simulink model "PI2GDL"  (R2018a)
settings: Solver=VariableStepAuto  StartTime=0.0  StopTime=200  RelTol=1e-3
values from neighbouring files (symbols this model uses):
  B = (T*tc)/(Ti)    (= 0.482939903103)    [Controlador2GDL.m]    (also in Examen2.m)
  k = 9.22    [Controlador2GDL.m]    (also in ControladorAlfaroPI1GDL_ControlEstricto.m; ControladorAlfaroPI1GDL_ControlSuave.m; Examen2.m)
  Kp = (a)/(k*(tc+to).^2)    [Controlador2GDL.m]    (also in ControladorAlfaroPI1GDL_ControlEstricto.m = 0.669122125129; ControladorAlfaroPI1GDL_ControlSuave.m = 0.469559386056; Examen2.m)
  L = 3.17    [Controlador2GDL.m]    (also in ControladorAlfaroPI1GDL_ControlEstricto.m; ControladorAlfaroPI1GDL_ControlSuave.m; Examen2.m)
  T = 34.31    [Controlador2GDL.m]    (also in ControladorAlfaroPI1GDL_ControlEstricto.m; ControladorAlfaroPI1GDL_ControlSuave.m; Examen2.m)
  Ti = T*(a/(1+to))    (= 14.2088072572)    [Controlador2GDL.m]    (also in ControladorAlfaroPI1GDL_ControlEstricto.m = 0.0291460215681; ControladorAlfaroPI1GDL_ControlSuave.m = 0.0291460215681; Examen2.m)
  Ts = 0.1    [Examen2.m]
settings Model: Creator=Rafael  LastModifiedBy=wivill
settings CodeAppCC: StateflowObjectComments=on

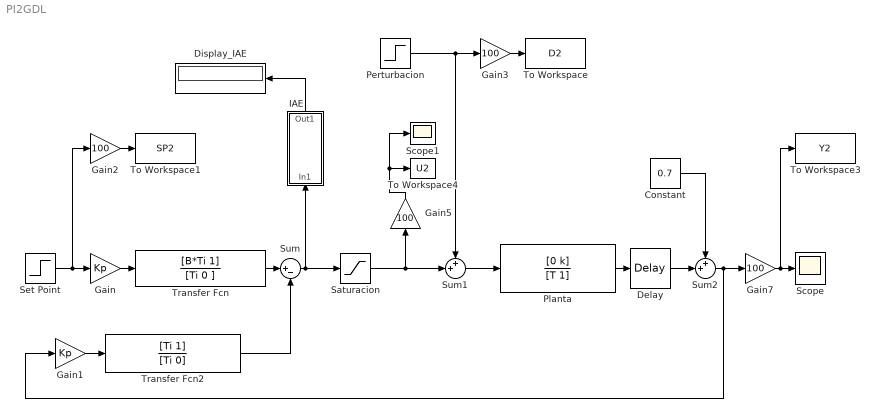
== system PI2GDL ==
  Constant : Constant  Value=0.7
  Delay : TransportDelay  DelayTime=L
  "Display_IAE " : Display
  Gain : Gain  Gain=Kp
  Gain1 : Gain  Gain=Kp
  Gain{2..3,5,7} (4 alike) : Gain  Gain=100
  IAE : Subsystem
      mask help:
      | IAE performacne index
      |
      | output = int |input| dt
      mask Display:
      | disp('IAE')
      | port_label('input',1,'e')
      | port_label('output',1,'iae')
  Perturbacion : Step  Time=75  After=-0.05  SampleTime=0
  Planta : TransferFcn  Numerator=[0 k]  Denominator=[T 1]
  "Saturacion " : Saturate  UpperLimit=1  LowerLimit=-0.1
  Scope : Scope
  Scope1 : Scope
  "Set Point " : Step  Time=0.1  Before=0.7  After=0.8  SampleTime=0
  Sum : Sum  Inputs=|+-
  Sum1 : Sum  Inputs=++|
  Sum2 : Sum  Inputs=++|
  To Workspace : ToWorkspace  VariableName=D2  SaveFormat=Timeseries  SampleTime=-1
  To Workspace1 : ToWorkspace  VariableName=SP2  SaveFormat=Timeseries  SampleTime=-1
  To Workspace3 : ToWorkspace  VariableName=Y2  SaveFormat=Timeseries  SampleTime=-1
  To Workspace4 : ToWorkspace  VariableName=U2  SaveFormat=Timeseries  SampleTime=Ts
  Transfer Fcn : TransferFcn  Numerator=[B*Ti 1]  Denominator=[Ti 0 ]
  Transfer Fcn2 : TransferFcn  Numerator=[Ti 1]  Denominator=[Ti 0]
  wires:
  Transfer Fcn/1 -> Sum/1
  Transfer Fcn2/1 -> Sum/2
  Planta/1 -> Delay/1
  Delay/1 -> Sum2/2
  Sum2/1 -> Gain7/1, Gain1/1
  Constant/1 -> Sum2/1
  Gain/1 -> Transfer Fcn/1
  Gain1/1 -> Transfer Fcn2/1
  IAE/1(Out1) -> "Display_IAE "/1
  Gain2/1 -> To Workspace1/1
  "Set Point "/1 -> Gain2/1, Gain/1
  "Saturacion "/1 -> Gain5/1, Sum1/2
  Sum/1 -> "Saturacion "/1, IAE/1(In1)
  Gain3/1 -> To Workspace/1
  Perturbacion/1 -> Gain3/1, Sum1/1
  Sum1/1 -> Planta/1
  Gain7/1 -> Scope/1, To Workspace3/1
  Gain5/1 -> To Workspace4/1, Scope1/1

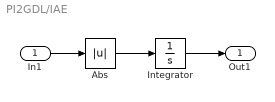
== system PI2GDL/IAE ==
  In1 : Inport
  Abs : Abs
  Integrator : Integrator
  Out1 : Outport
  wires:
  In1/1 -> Abs/1
  Integrator/1 -> Out1/1
  Abs/1 -> Integrator/1
